simulink model "quest2"  (R2015a)
settings: Solver=ode3  StartTime=0.0  StopTime=20  FixedStep=0.01  RelTol=1e-3
libraries: simulink x1
settings Model: CovModelRefEnable=off  Creator=Subodh  LastModifiedBy=smishra
settings DataIOCC: SaveFormat=Dataset
settings HardwareCC: ProdBitPerPointer=64  ProdLargestAtomicFloat=Float  ProdIntDivRoundTo=Zero  ProdEndianess=LittleEndian  ProdHWDeviceType=Specified
settings GRTTargetCC: GeneratePreprocessorConditionals=Use local settings

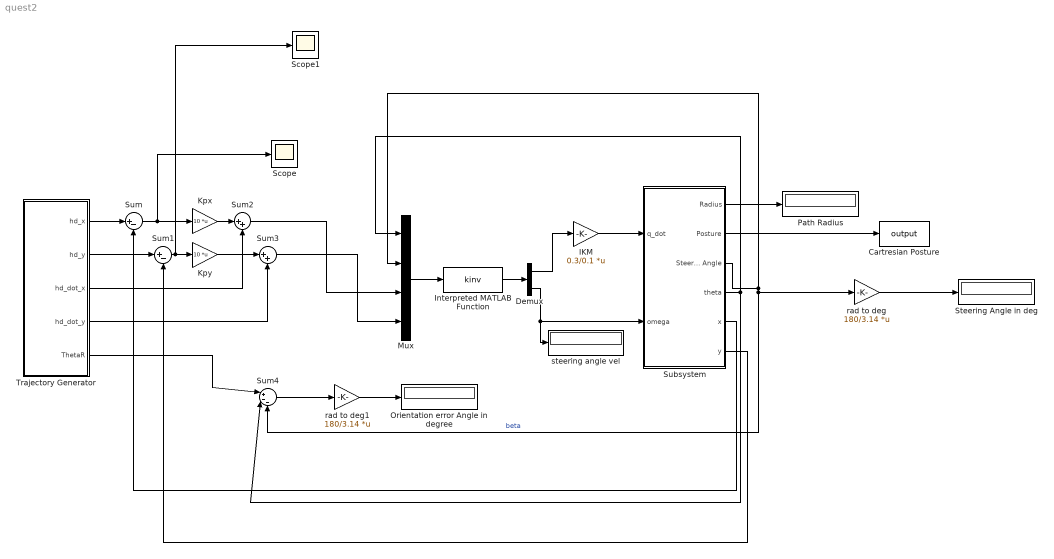
== system quest2 ==
  Cartresian Posture : ToWorkspace  VariableName=output  SampleTime=-1
  Demux : Demux  Outputs=2
  IKM : Gain  Gain=0.3/0.1  Multiplication=Matrix(K*u)
  Interpreted MATLAB Function : MATLABFcn  MATLABFcn=kinv  OutputDimensions=2
  Kpx : Gain  Gain=10  Multiplication=Matrix(K*u)
  Kpy : Gain  Gain=10  Multiplication=Matrix(K*u)
  Mux : Mux
  Orientation error Angle in degree : Display
  Path Radius : Display
  Scope : Scope
  Scope1 : Scope
  Steering Angle in deg : Display
  Subsystem : Subsystem
  Sum : Sum  Inputs=|+-
  Sum1 : Sum  Inputs=|+-
  Sum2 : Sum  Inputs=|++
  Sum3 : Sum  Inputs=|++
  Sum4 : Sum  Inputs=|+--
  Trajectory Generator : Subsystem
  rad to deg : Gain  Gain=180/3.14  Multiplication=Matrix(K*u)
  rad to deg1 : Gain  Gain=180/3.14  Multiplication=Matrix(K*u)
  steering angle vel : Display
  wires:
  Subsystem/1("Radius ") -> Path Radius/1
  Subsystem/2(Posture) -> Cartresian Posture/1
  Subsystem/3(Steering Angle) -> rad to deg/1, Sum4/3, Mux/2  "beta"
  IKM/1 -> Subsystem/1(q_dot)
  Mux/1 -> Interpreted MATLAB Function/1
  Subsystem/4(theta) -> Mux/1, Sum4/2
  Trajectory Generator/1(hd_x) -> Sum/1
  Subsystem/5(x) -> Sum/2
  Trajectory Generator/2(hd_y) -> Sum1/1
  Subsystem/6(y) -> Sum1/2
  Sum/1 -> Scope/1, Kpx/1
  Kpx/1 -> Sum2/1
  Trajectory Generator/3(hd_dot_x) -> Sum2/2
  Sum1/1 -> Scope1/1, Kpy/1
  Kpy/1 -> Sum3/1
  Trajectory Generator/4(hd_dot_y) -> Sum3/2
  Sum2/1 -> Mux/3
  Sum3/1 -> Mux/4
  Interpreted MATLAB Function/1 -> Demux/1
  Demux/1 -> IKM/1
  Demux/2 -> Subsystem/2(omega), steering angle vel/1
  Trajectory Generator/5(ThetaR) -> Sum4/1
  rad to deg/1 -> Steering Angle in deg/1
  Sum4/1 -> rad to deg1/1
  rad to deg1/1 -> Orientation error Angle in degree/1

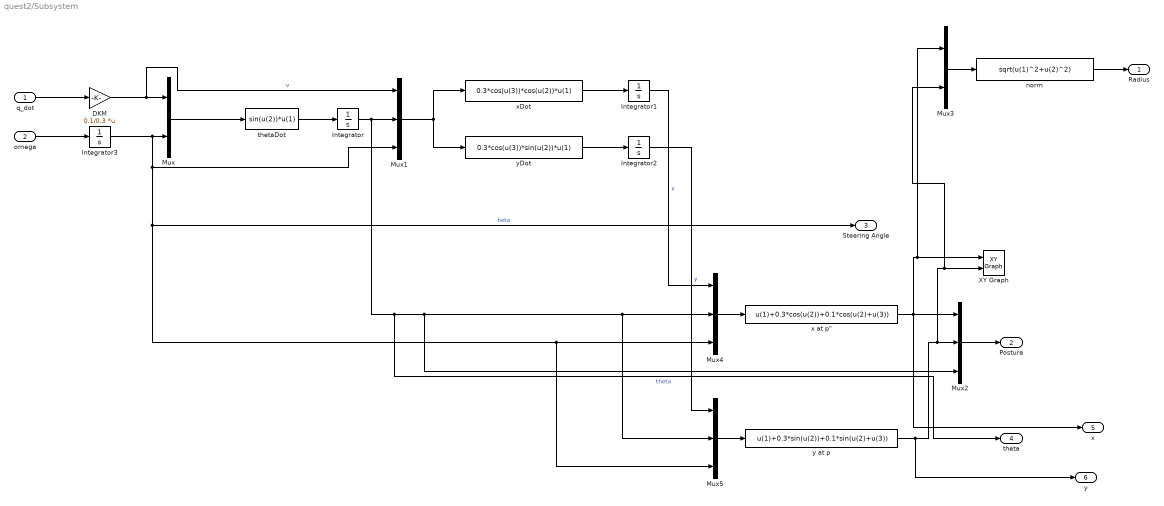
== system quest2/Subsystem ==
  q_dot : Inport
  omega : Inport  Port=2
  DKM : Gain  Gain=0.1/0.3  Multiplication=Matrix(K*u)
  Integrator{,1..3} (4 alike) : Integrator
  Mux : Mux  Inputs=2
  Mux{1..2,4..5} (4 alike) : Mux  Inputs=3
  Mux3 : Mux  Inputs=2
  XY Graph : simulink/Sinks/XY Graph  xmin=-3  xmax=3  ymin=-3  ymax=3  st=-1
  norm : Fcn  Expr=sqrt(u(1)^2+u(2)^2)
  thetaDot : Fcn  Expr=sin(u(2))*u(1)
  "x at p\"" : Fcn  Expr=u(1)+0.3*cos(u(2))+0.1*cos(u(2)+u(3))
  xDot : Fcn  Expr=0.3*cos(u(3))*cos(u(2))*u(1)
  y at p : Fcn  Expr=u(1)+0.3*sin(u(2))+0.1*sin(u(2)+u(3))
  yDot : Fcn  Expr=0.3*cos(u(3))*sin(u(2))*u(1)
  "Radius " : Outport
  Posture : Outport  Port=2
  Steering Angle : Outport  Port=3
  theta : Outport  Port=4
  x : Outport  Port=5
  y : Outport  Port=6
  wires:
  Mux/1 -> thetaDot/1
  Integrator/1 -> theta/1, Mux2/3, Mux5/2, Mux4/2, Mux1/2  "theta"
  xDot/1 -> Integrator1/1
  Mux3/1 -> norm/1
  thetaDot/1 -> Integrator/1
  Mux1/1 -> xDot/1, yDot/1
  yDot/1 -> Integrator2/1
  Integrator1/1 -> Mux4/1  "x"
  Integrator2/1 -> Mux5/1  "y"
  Integrator3/1 -> Mux5/3, Mux4/3, Steering Angle/1, Mux1/3, Mux/2  "beta"
  norm/1 -> "Radius "/1
  q_dot/1 -> DKM/1
  DKM/1 -> Mux1/1, Mux/1  "v"
  Mux4/1 -> "x at p\""/1
  Mux5/1 -> y at p/1
  "x at p\""/1 -> x/1, Mux3/1, XY Graph/1, Mux2/1
  y at p/1 -> y/1, Mux3/2, XY Graph/2, Mux2/2
  Mux2/1 -> Posture/1
  omega/1 -> Integrator3/1

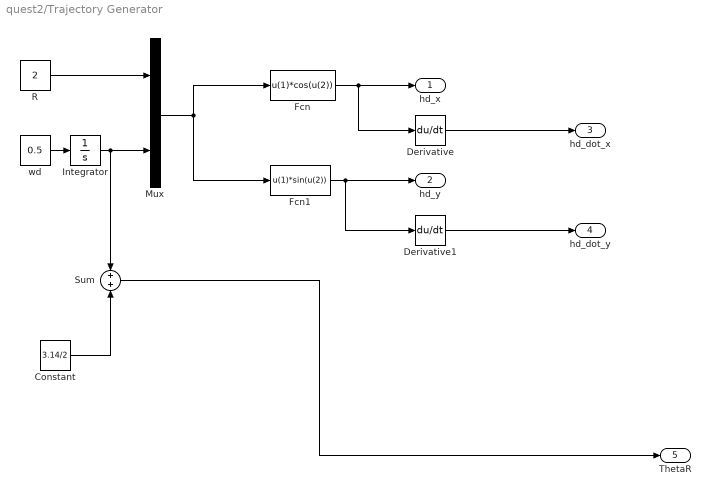
== system quest2/Trajectory Generator ==
  Constant : Constant  Value=3.14/2
  Derivative : Derivative
  Derivative1 : Derivative
  Fcn : Fcn  Expr=u(1)*cos(u(2))
  Fcn1 : Fcn  Expr=u(1)*sin(u(2))
  Integrator : Integrator
  Mux : Mux  Inputs=2
  R : Constant  Value=2
  Sum : Sum
  wd : Constant  Value=0.5
  hd_x : Outport
  hd_y : Outport  Port=2
  hd_dot_x : Outport  Port=3
  hd_dot_y : Outport  Port=4
  ThetaR : Outport  Port=5
  wires:
  Fcn/1 -> Derivative/1, hd_x/1
  Fcn1/1 -> Derivative1/1, hd_y/1
  Mux/1 -> Fcn1/1, Fcn/1
  R/1 -> Mux/1
  wd/1 -> Integrator/1
  Derivative/1 -> hd_dot_x/1
  Derivative1/1 -> hd_dot_y/1
  Constant/1 -> Sum/2
  Integrator/1 -> Sum/1, Mux/2
  Sum/1 -> ThetaR/1
